simulink model "auxx"  (R2019a)
settings: Solver=VariableStepAuto  StartTime=0.0  StopTime=10.0  RelTol=1e-3
values from neighbouring files (symbols this model uses):
  A_AA = [ybb  yp+w0/u0 yr-1 g*ctt0/u0 ... (first row only)    [P1.m]    (also in P2.m; P3.m; P3_F.m; P3_serv.m)
  B = [0    ydr ... (first row only)    [P1.m]    (also in P2.m; P3.m; P3_F.m; P3_serv.m)
  bb_ref = 3    [P3.m]    (also in P3_F.m = 0.8; P3_serv.m = 0.8; P3_test.m; P4_F.m = 0.8)
  bb_stept = 10    [P3.m]    (also in P3_F.m; P3_serv.m; P3_test.m; P4_F.m)
  C = eye(4)    [P2.m]    (also in P3.m; P3_F.m; P3_serv.m; P3_test.m)
  D = zeros(4,2)    [P2.m]    (also in P3.m; P3_F.m; P3_serv.m; P3_test.m)
  damax = [-18 18]    [P1.m]    (also in P2.m; P3.m; P3_F.m; P3_serv.m)
  deg = pi/180    (= 0.0174532925199)    [P1.m]    (also in P2.m; P3.m; P3_F.m; P3_serv.m)
  drmax = [-23 23]    [P1.m]    (also in P2.m; P3.m; P3_F.m; P3_serv.m)
  F = (CC*dcgain)^(-1)    [P3_F.m]    (also in P3_test.m; P4_F.m; P5.m; P5_F.m)
  g = 9.81    [P1.m]    (also in P2.m; P3.m; P3_F.m; P3_serv.m)
  K_lqr = lqr(A2_AA,B2,Q,R)    [P3.m]    (also in P3_F.m = lqr(A_AA,B,Q,R); P3_serv.m; P3_test.m = lqr(A_AA,B,Q,R); P4_F.m = lqr(A_AA,B,Q,R))
  K_psi = 2.49    [P5_F.m]    (also in P5_F_Delta.m; auxxx.m)
  phi_ref = 8    [P3.m]    (also in P3_F.m = 15; P3_serv.m; P3_test.m; P4_F.m = 22)
  phi_stept = 50    [P3.m]    (also in P3_F.m; P3_serv.m; P3_test.m; P4_F.m)
  u0 = u0*knot2ms    (= 134.475777662)    [P1.m]    (also in P2.m; P3.m; P3_F.m; P3_serv.m)
libraries: simulink x7
settings Model: Creator=User  LastModifiedBy=User
settings DebuggingCC: SFMachineParentedDataDiag=error

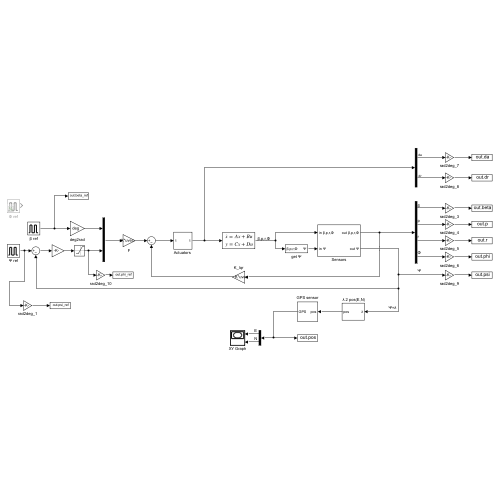
[thumbnail: Simulink's stored preview of the top-level diagram]
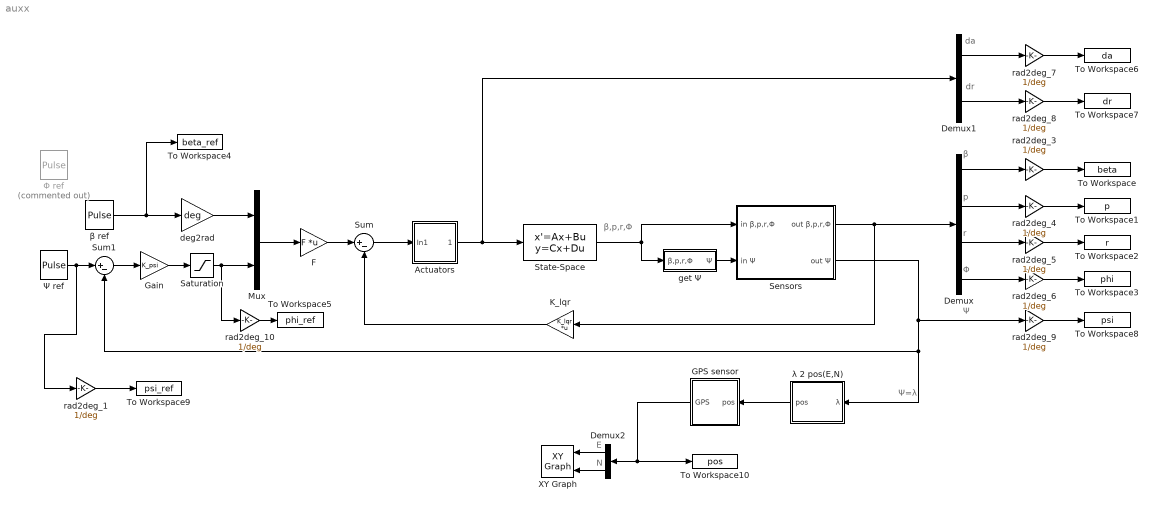
== system auxx ==
  note: r
  note: β
  note: β,p,r,Φ
  note: Ψ
  note: da
  note: Φ
  note: E
  note: dr
  note: p
  note: Ψ=λ
  note: N
  " λ 2 pos(E,N)" : Subsystem
  "Actuators " : Subsystem
  Demux : Demux
  Demux1 : Demux  Outputs=2
  Demux2 : Demux  Outputs=2
  F : Gain  Gain=F  Multiplication=Matrix(K*u) (u vector)
  GPS sensor : Subsystem
  Gain : Gain  Gain=K_psi
  K_lqr : Gain  Gain=K_lqr  Multiplication=Matrix(K*u) (u vector)
  Mux : Mux  Inputs=2
  Saturation : Saturate  UpperLimit=30*deg  LowerLimit=-30*deg
  Sensors : Subsystem
  State-Space : StateSpace  A=A_AA  B=B  C=C  D=D  InitialCondition=0
  Sum : Sum  Inputs=|+-
  Sum1 : Sum  Inputs=|+-
  To Workspace : ToWorkspace  VariableName=beta  SaveFormat=Timeseries  SampleTime=-1
  To Workspace1 : ToWorkspace  VariableName=p  SaveFormat=Timeseries  SampleTime=-1
  To Workspace10 : ToWorkspace  VariableName=pos  SaveFormat=Timeseries  SampleTime=-1
  To Workspace2 : ToWorkspace  VariableName=r  SaveFormat=Timeseries  SampleTime=-1
  To Workspace3 : ToWorkspace  VariableName=phi  SaveFormat=Timeseries  SampleTime=-1
  To Workspace4 : ToWorkspace  VariableName=beta_ref  SaveFormat=Timeseries  SampleTime=-1
  To Workspace5 : ToWorkspace  VariableName=phi_ref  SaveFormat=Timeseries  SampleTime=-1
  To Workspace6 : ToWorkspace  VariableName=da  SaveFormat=Timeseries  SampleTime=-1
  To Workspace7 : ToWorkspace  VariableName=dr  SaveFormat=Timeseries  SampleTime=-1
  To Workspace8 : ToWorkspace  VariableName=psi  SaveFormat=Timeseries  SampleTime=-1
  To Workspace9 : ToWorkspace  VariableName=psi_ref  SaveFormat=Timeseries  SampleTime=-1
  XY Graph : simulink/Sinks/XY Graph  xmin=-1  xmax=1  ymin=-1  ymax=1  st=-1
  deg2rad : Gain  Gain=deg
  get Ψ : Subsystem
  rad2deg_{1,3..10} (9 alike) : Gain  Gain=1/deg
  Φ ref : DiscretePulseGenerator  Commented=on  PulseType=Time based  Amplitude=phi_ref  Period=100  PulseWidth=20  PhaseDelay=phi_stept
  Ψ ref : DiscretePulseGenerator  PulseType=Time based  Amplitude=10*deg  Period=100  PulseWidth=20  PhaseDelay=20
  β ref : DiscretePulseGenerator  PulseType=Time based  Amplitude=bb_ref  Period=100  PulseWidth=20  PhaseDelay=bb_stept
  wires:
  Sum1/1 -> Gain/1
  rad2deg_10/1 -> To Workspace5/1
  rad2deg_8/1 -> To Workspace7/1
  Demux/4 -> rad2deg_6/1
  GPS sensor/1(GPS) -> Demux2/1, To Workspace10/1
  Sensors/1(out β,p,r,Φ) -> K_lqr/1, Demux/1
  deg2rad/1 -> Mux/1
  Saturation/1 -> Mux/2, rad2deg_10/1
  rad2deg_7/1 -> To Workspace6/1
  " λ 2 pos(E,N)"/1(pos) -> GPS sensor/1(pos)
  Demux2/1 -> XY Graph/1
  Demux2/2 -> XY Graph/2
  rad2deg_4/1 -> To Workspace1/1
  Sensors/2(out Ψ) -> Sum1/2, " λ 2 pos(E,N)"/1(" λ"), rad2deg_9/1
  rad2deg_5/1 -> To Workspace2/1
  rad2deg_3/1 -> To Workspace/1
  "Actuators "/1(Out1) -> Demux1/1, State-Space/1
  F/1 -> Sum/1
  β ref/1 -> To Workspace4/1, deg2rad/1
  get Ψ/1(Ψ) -> Sensors/2(in Ψ)
  Gain/1 -> Saturation/1
  rad2deg_9/1 -> To Workspace8/1
  Demux/2 -> rad2deg_4/1
  Sum/1 -> "Actuators "/1(In1)
  Demux1/2 -> rad2deg_8/1
  rad2deg_6/1 -> To Workspace3/1
  State-Space/1 -> Sensors/1(in β,p,r,Φ), get Ψ/1(β,p,r,Φ)
  Demux1/1 -> rad2deg_7/1
  Demux/3 -> rad2deg_5/1
  K_lqr/1 -> Sum/2
  Mux/1 -> F/1
  Demux/1 -> rad2deg_3/1
  Ψ ref/1 -> rad2deg_1/1, Sum1/1
  rad2deg_1/1 -> To Workspace9/1

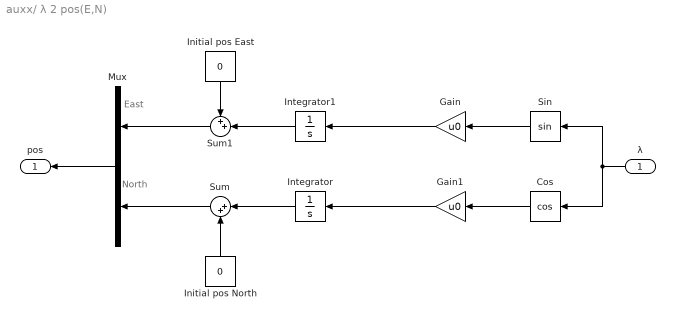
== system auxx/ λ 2 pos(E,N) ==
  note: North
  note: East
  " λ" : Inport
  Cos : Trigonometry  Operator=cos
  Gain : Gain  Gain=u0
  Gain1 : Gain  Gain=u0
  Initial pos East : Constant  Value=0
  Initial pos North : Constant  Value=0
  Integrator : Integrator
  Integrator1 : Integrator
  Mux : Mux  Inputs=2
  Sin : Trigonometry
  Sum : Sum  Inputs=|++
  Sum1 : Sum  Inputs=++|
  pos : Outport
  wires:
  Mux/1 -> pos/1
  " λ"/1 -> Cos/1, Sin/1
  Sin/1 -> Gain/1
  Cos/1 -> Gain1/1
  Gain/1 -> Integrator1/1
  Gain1/1 -> Integrator/1
  Integrator/1 -> Sum/1
  Sum/1 -> Mux/2
  Integrator1/1 -> Sum1/2
  Sum1/1 -> Mux/1
  Initial pos East/1 -> Sum1/1
  Initial pos North/1 -> Sum/2

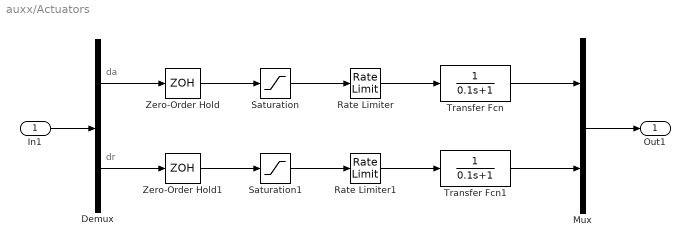
== system auxx/Actuators  ==
  note: da
  note: dr
  In1 : Inport
  Demux : Demux  Outputs=2
  Mux : Mux  Inputs=2
  Rate Limiter : RateLimiter  RisingSlewLimit=60*deg  FallingSlewLimit=-60*deg  SampleTimeMode=inherited
  Rate Limiter1 : RateLimiter  RisingSlewLimit=60*deg  FallingSlewLimit=-60*deg  SampleTimeMode=inherited
  Saturation : Saturate  UpperLimit=damax(2) * deg  LowerLimit=damax(1) * deg
  Saturation1 : Saturate  UpperLimit=drmax(2) * deg  LowerLimit=drmax(1) * deg
  Transfer Fcn : TransferFcn  Denominator=[0.1 1]
  Transfer Fcn1 : TransferFcn  Denominator=[0.1 1]
  Zero-Order Hold : ZeroOrderHold  SampleTime=0.025
  Zero-Order Hold1 : ZeroOrderHold  SampleTime=0.025
  Out1 : Outport
  wires:
  In1/1 -> Demux/1
  Demux/1 -> Zero-Order Hold/1
  Demux/2 -> Zero-Order Hold1/1
  Zero-Order Hold/1 -> Saturation/1
  Zero-Order Hold1/1 -> Saturation1/1
  Saturation/1 -> Rate Limiter/1
  Saturation1/1 -> Rate Limiter1/1
  Rate Limiter/1 -> Transfer Fcn/1
  Rate Limiter1/1 -> Transfer Fcn1/1
  Transfer Fcn/1 -> Mux/1
  Transfer Fcn1/1 -> Mux/2
  Mux/1 -> Out1/1

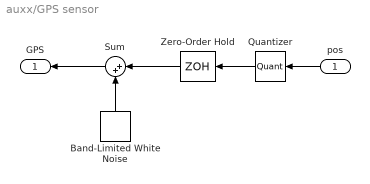
== system auxx/GPS sensor ==
  pos : Inport
  Band-Limited White Noise : simulink/Sources/Band-Limited White Noise  Cov=[6^2/1]  Ts=1  seed=[23341]
  Quantizer : Quantizer
  Sum : Sum  Inputs=|++
  Zero-Order Hold : ZeroOrderHold
  GPS : Outport
  wires:
  Band-Limited White Noise/1 -> Sum/2
  pos/1 -> Quantizer/1
  Quantizer/1 -> Zero-Order Hold/1
  Zero-Order Hold/1 -> Sum/1
  Sum/1 -> GPS/1

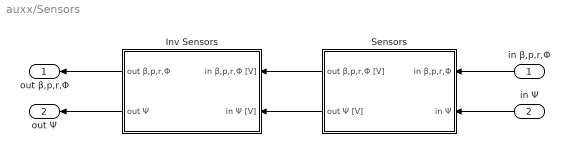
== system auxx/Sensors ==
  in β,p,r,Φ : Inport
  in Ψ : Inport  Port=2
  Inv Sensors : Subsystem
  Sensors : Subsystem
  out β,p,r,Φ : Outport
  out Ψ : Outport  Port=2
  wires:
  Sensors/1(out β,p,r,Φ [V]) -> Inv Sensors/1(in β,p,r,Φ [V])
  Inv Sensors/1(out β,p,r,Φ) -> out β,p,r,Φ/1
  in β,p,r,Φ/1 -> Sensors/1(in β,p,r,Φ)
  in Ψ/1 -> Sensors/2(in Ψ)
  Sensors/2(out Ψ [V]) -> Inv Sensors/2(in Ψ [V])
  Inv Sensors/2(out Ψ) -> out Ψ/1

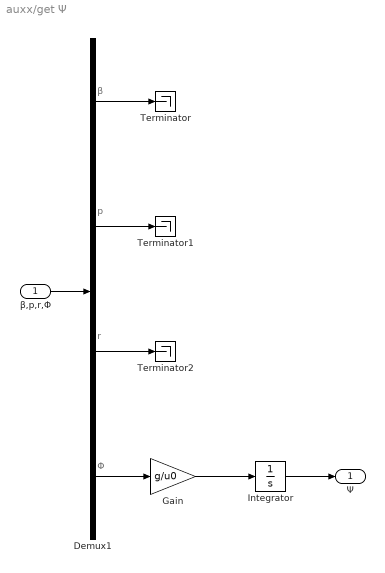
== system auxx/get Ψ ==
  note: Φ
  note: r
  note: p
  note: β
  β,p,r,Φ : Inport
  Demux1 : Demux
  Gain : Gain  Gain=g/u0
  Integrator : Integrator
  Terminator : Terminator
  Terminator1 : Terminator
  Terminator2 : Terminator
  Ψ : Outport  VectorParamsAs1DForOutWhenUnconnected=off
  wires:
  β,p,r,Φ/1 -> Demux1/1
  Demux1/1 -> Terminator/1
  Demux1/2 -> Terminator1/1
  Demux1/3 -> Terminator2/1
  Demux1/4 -> Gain/1
  Gain/1 -> Integrator/1
  Integrator/1 -> Ψ/1

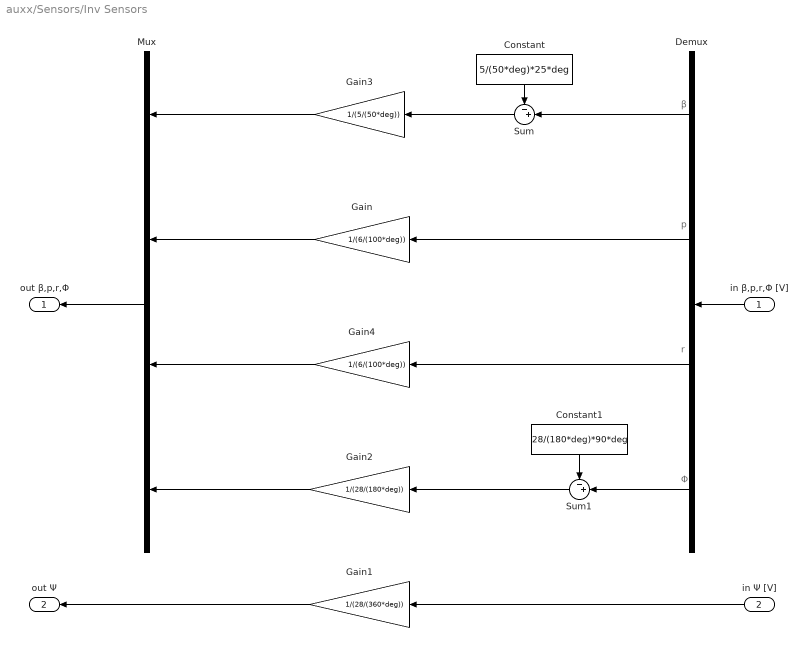
== system auxx/Sensors/Inv Sensors ==
  note: p
  note: β
  note: Φ
  note: r
  in β,p,r,Φ [V] : Inport
  in Ψ [V] : Inport  Port=2
  Constant : Constant  Value=5/(50*deg)*25*deg
  Constant1 : Constant  Value=28/(180*deg)*90*deg
  Demux : Demux
  Gain : Gain  Gain=1/(6/(100*deg))
  Gain1 : Gain  Gain=1/(28/(360*deg))
  Gain2 : Gain  Gain=1/(28/(180*deg))
  Gain3 : Gain  Gain=1/(5/(50*deg))
  Gain4 : Gain  Gain=1/(6/(100*deg))
  Mux : Mux
  Sum : Sum  Inputs=-+|
  Sum1 : Sum  Inputs=-+|
  out β,p,r,Φ : Outport
  out Ψ : Outport  Port=2  VectorParamsAs1DForOutWhenUnconnected=off
  wires:
  Demux/4 -> Sum1/2
  Demux/2 -> Gain/1
  Mux/1 -> out β,p,r,Φ/1
  in β,p,r,Φ [V]/1 -> Demux/1
  Sum1/1 -> Gain2/1
  Gain3/1 -> Mux/1
  Constant/1 -> Sum/1
  Demux/1 -> Sum/2
  Sum/1 -> Gain3/1
  Demux/3 -> Gain4/1
  Constant1/1 -> Sum1/1
  Gain2/1 -> Mux/4
  Gain4/1 -> Mux/3
  Gain/1 -> Mux/2
  Gain1/1 -> out Ψ/1
  in Ψ [V]/1 -> Gain1/1

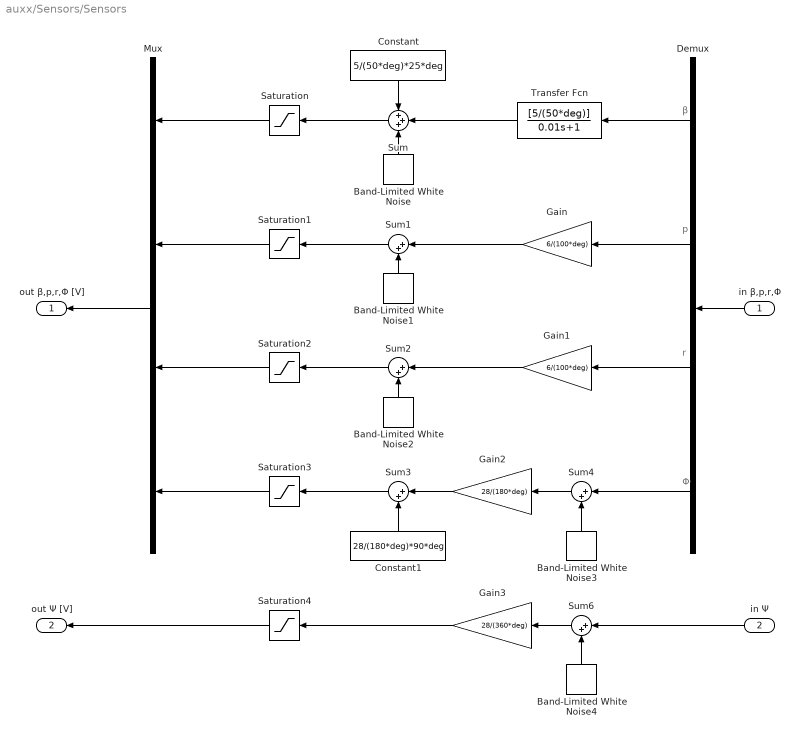
== system auxx/Sensors/Sensors ==
  note: β
  note: p
  note: r
  note: Φ
  in β,p,r,Φ : Inport
  in Ψ : Inport  Port=2
  Band-Limited White Noise : simulink/Sources/Band-Limited White Noise  Cov=[0.005^2/40]  Ts=0.025  seed=[23341]
  Band-Limited White Noise1 : simulink/Sources/Band-Limited White Noise  Cov=[0.002^2/40]  Ts=0.025  seed=[23341]
  Band-Limited White Noise2 : simulink/Sources/Band-Limited White Noise  Cov=[0.002^2/40]  Ts=0.025  seed=[23341]
  Band-Limited White Noise3 : simulink/Sources/Band-Limited White Noise  Cov=[(0.25*deg)^2/40]  Ts=0.025  seed=[23341]
  Band-Limited White Noise4 : simulink/Sources/Band-Limited White Noise  Cov=[(1.5*deg)^2/40]  Ts=0.025  seed=[23341]
  Constant : Constant  Value=5/(50*deg)*25*deg
  Constant1 : Constant  Value=28/(180*deg)*90*deg
  Demux : Demux
  Gain : Gain  Gain=6/(100*deg)
  Gain1 : Gain  Gain=6/(100*deg)
  Gain2 : Gain  Gain=28/(180*deg)
  Gain3 : Gain  Gain=28/(360*deg)
  Mux : Mux
  Saturation : Saturate  UpperLimit=5  LowerLimit=0
  Saturation1 : Saturate  UpperLimit=3  LowerLimit=-3
  Saturation2 : Saturate  UpperLimit=3  LowerLimit=-3
  Saturation3 : Saturate  UpperLimit=28  LowerLimit=0
  Saturation4 : Saturate  UpperLimit=28  LowerLimit=0
  Sum : Sum  Inputs=+++
  Sum{1..4,6} (5 alike) : Sum  Inputs=|++
  Transfer Fcn : TransferFcn  Numerator=[5/(50*deg)]  Denominator=[0.01 1]
  out β,p,r,Φ [V] : Outport
  out Ψ [V] : Outport  Port=2  VectorParamsAs1DForOutWhenUnconnected=off
  wires:
  in β,p,r,Φ/1 -> Demux/1
  Demux/1 -> Transfer Fcn/1
  Transfer Fcn/1 -> Sum/2
  Constant/1 -> Sum/1
  Band-Limited White Noise/1 -> Sum/3
  Sum/1 -> Saturation/1
  Saturation/1 -> Mux/1
  Mux/1 -> out β,p,r,Φ [V]/1
  Demux/2 -> Gain/1
  Gain/1 -> Sum1/1
  Band-Limited White Noise1/1 -> Sum1/2
  Sum1/1 -> Saturation1/1
  Saturation1/1 -> Mux/2
  Demux/3 -> Gain1/1
  Sum2/1 -> Saturation2/1
  Band-Limited White Noise2/1 -> Sum2/2
  Gain1/1 -> Sum2/1
  Saturation2/1 -> Mux/3
  Sum3/1 -> Saturation3/1
  Constant1/1 -> Sum3/2
  Gain2/1 -> Sum3/1
  Sum4/1 -> Gain2/1
  Demux/4 -> Sum4/1
  Saturation3/1 -> Mux/4
  Band-Limited White Noise3/1 -> Sum4/2
  Sum6/1 -> Gain3/1
  Band-Limited White Noise4/1 -> Sum6/2
  Gain3/1 -> Saturation4/1
  in Ψ/1 -> Sum6/1
  Saturation4/1 -> out Ψ [V]/1
